simulink model "redundancy"  (R2020b)
settings: Solver=ode15s  StartTime=0.0  StopTime=T  MaxStep=0.01  RelTol=1e-3
values from neighbouring files (symbols this model uses):
  a1A = L1    (= 0.35)    [forward_kinematics_computation.m]
  a1B = L1    (= 0.35)    [forward_kinematics_computation.m]
  a2A = L2    (= 0.305)    [forward_kinematics_computation.m]
  a2B = L2    (= 0.305)    [forward_kinematics_computation.m]
  a3A = L3    (= 0.2662)    [forward_kinematics_computation.m]
  a3B = L3    (= 0.2662)    [forward_kinematics_computation.m]
  D = 1.047    [forward_kinematics_computation.m]
  dq0 = [0 0 0 0 0 0]'    [sim_redundancy.m]
  friction = [fv1p fv2p fv1A fv2A fv3A fv1B fv2B fv3B]    [sim_redundancy.m]
  g = [0 -g0 0]'    [sim_redundancy.m]
  Gd = diag([1000 1000 1000 1000 1000])    [sim_redundancy.m]
  Gd_nullspace = 10*eye(6)    [sim_redundancy.m]
  Gp = diag([3000 3000 3000 3000 1000])    [sim_redundancy.m]
  Gp_nullspace = 10*eye(6)    [sim_redundancy.m]
  info = struct('n_joints', n_joints,                'n_links', n_links,                'n_ee', n_ee,                'current_frame_index',    [1  2 3 4 5 6 7  8 9 10],                'previous_frame_index',   [0  1 2 3 4 2 6  7 5  8],                'next_frame_index',       [2 36 4 5 9 7 8 10 0  0],                'next_frame_type',        [0  1 0 0 0 0 0  0 0  0],                'previous_joint_index',  ...(+449 chars)    [sim_redundancy.m]
  Kd = 20*eye(6)    [sim_redundancy.m]
  Kp = 10*eye(6)    [sim_redundancy.m]
  L = 3.16 + 0.126    (= 3.286)    [forward_kinematics_computation.m]
  l1A = a1A/2    (= 0.175)    [forward_kinematics_computation.m]
  l1B = a1B/2    (= 0.175)    [forward_kinematics_computation.m]
  l2A = a2A/2    (= 0.1525)    [forward_kinematics_computation.m]
  l2B = a2B/2    (= 0.1525)    [forward_kinematics_computation.m]
  l3A = a3A/2    (= 0.1331)    [forward_kinematics_computation.m]
  l3B = a3B/2    (= 0.1331)    [forward_kinematics_computation.m]
  offA = -0.19    [forward_kinematics_computation.m]
  offB = 0.19    [forward_kinematics_computation.m]
  prova = 2    [sim_redundancy.m]
  q0 = [th1A_0 th2A_0 th3A_0 th1B_0 th2B_0 th3B_0]'    [sim_redundancy.m]
  qr = [0 -pi/3 pi/4 0 pi/4 pi/8]    [sim_redundancy.m]
  qr_ddot = zeros(1,6)    [sim_redundancy.m]
  qr_dot = zeros(1,6)    [sim_redundancy.m]
  th1A_0 = -pi/6    (= -0.523598775598)    [sim_redundancy.m]
  th1B_0 = pi/6    (= 0.523598775598)    [sim_redundancy.m]
  th2A_0 = pi/6    (= 0.523598775598)    [sim_redundancy.m]
  th2B_0 = -pi/6    (= -0.523598775598)    [sim_redundancy.m]
  th3A_0 = pi/6    (= 0.523598775598)    [sim_redundancy.m]
  th3B_0 = -pi/6    (= -0.523598775598)    [sim_redundancy.m]
  tipo_controllo = 1    [sim_redundancy.m]
  tipo_minimizzazione = 4    [sim_redundancy.m]
  x_ref = [-0.25 -0.8 0.19 -0.9 0]    [sim_redundancy.m]
  xddot_ref = [0 0 0 0 0]    [sim_redundancy.m]
  xdot_ref = [0 0 0 0 0]    [sim_redundancy.m]
undefined symbols (not defined in the file or in its folder): fv0, fv1A, fv1B, fv2A, fv2B, fv3A, fv3B, g0, Il1Azz, Il1Bzz, Il2Azz, Il2Bzz, Il3Azz, Il3Bzz, m_cables, m_crane, m_platform, ml1A, ml1B, ml2A, ml2B, ml3A, ml3B, X, Y, Z
libraries: sm_lib x137, nesl_utility x31
(part 5 of 5)

== matlab function redundancy/CLIK 2/Ja_dot*qd ==
  data: q input; qd input; out output; a1A parameter; a2A parameter; a3A parameter; a1B parameter; a2B parameter; a3B parameter; offA parameter; offB parameter; ml1A parameter; ml2A parameter; ml3A parameter; ml1B parameter; ml2B parameter; ml3B parameter; l1A parameter; l2A parameter; l3A parameter; l1B parameter; l2B parameter; l3B parameter
function out = fcn(q, qd, ...
                  a1A, a2A, a3A, a1B, a2B, a3B, offA, offB, ...
                  ml1A, ml2A, ml3A, ml1B, ml2B, ml3B, ...
                  l1A, l2A, l3A, l1B, l2B, l3B)

% Input
th1A = q(1);
th2A = q(2);
th3A = q(3);
th1B = q(4);
th2B = q(5);
th3B = q(6);
dth1A = qd(1);
dth2A = qd(2);
dth3A = qd(3);
dth1B = qd(4);
dth2B = qd(5);
dth3B = qd(6);

% Derivata dello Jacobiano
Jad = [                                                                                                                                  - a1A*dth1A*sin(th1A) - a3A*sin(th1A + th2A + th3A)*(dth1A + dth2A + dth3A) - a2A*sin(th1A + th2A)*(dth1A + dth2A),                                                                                - a3A*sin(th1A + th2A + th3A)*(dth1A + dth2A + dth3A) - a2A*sin(th1A + th2A)*(dth1A + dth2A),                                   -a3A*sin(th1A + th2A + th3A)*(dth1A + dth2A + dth3A),                                                                                                                                                                                                                                                    0,                                                                                                                                                                           0,                                                                                      0;
                                                                                                                                           a3A*cos(th1A + th2A + th3A)*(dth1A + dth2A + dth3A) + a2A*cos(th1A + th2A)*(dth1A + dth2A) + a1A*dth1A*cos(th1A),                                                                                  a3A*cos(th1A + th2A + th3A)*(dth1A + dth2A + dth3A) + a2A*cos(th1A + th2A)*(dth1A + dth2A),                                    a3A*cos(th1A + th2A + th3A)*(dth1A + dth2A + dth3A),                                                                                                                                                                                                                                                    0,                                                                                                                                                                           0,                                                                                      0;
                                                                                                                                                                                                                                                          0,                                                                                                                                                                           0,                                                                                      0,                                                                                                                                   - a1B*dth1B*sin(th1B) - a3B*sin(th1B + th2B + th3B)*(dth1B + dth2B + dth3B) - a2B*sin(th1B + th2B)*(dth1B + dth2B),                                                                                - a3B*sin(th1B + th2B + th3B)*(dth1B + dth2B + dth3B) - a2B*sin(th1B + th2B)*(dth1B + dth2B),                                   -a3B*sin(th1B + th2B + th3B)*(dth1B + dth2B + dth3B);
                                                                                                                                                                                                                                                          0,                                                                                                                                                                           0,                                                                                      0,                                                                                                                                     a3B*cos(th1B + th2B + th3B)*(dth1B + dth2B + dth3B) + a2B*cos(th1B + th2B)*(dth1B + dth2B) + a1B*dth1B*cos(th1B),                                                                                  a3B*cos(th1B + th2B + th3B)*(dth1B + dth2B + dth3B) + a2B*cos(th1B + th2B)*(dth1B + dth2B),                                    a3B*cos(th1B + th2B + th3B)*(dth1B + dth2B + dth3B);
       -(ml3A*(a1A*dth1A*sin(th1A) + l3A*sin(th1A + th2A + th3A)*(dth1A + dth2A + dth3A) + a2A*sin(th1A + th2A)*(dth1A + dth2A)) + ml2A*(a1A*dth1A*sin(th1A) + l2A*sin(th1A + th2A)*(dth1A + dth2A)) + dth1A*l1A*ml1A*sin(th1A))/(2*ml1A + 2*ml2A + 2*ml3A), -(ml3A*(l3A*sin(th1A + th2A + th3A)*(dth1A + dth2A + dth3A) + a2A*sin(th1A + th2A)*(dth1A + dth2A)) + l2A*ml2A*sin(th1A + th2A)*(dth1A + dth2A))/(2*ml1A + 2*ml2A + 2*ml3A), -(l3A*ml3A*sin(th1A + th2A + th3A)*(dth1A + dth2A + dth3A))/(2*ml1A + 2*ml2A + 2*ml3A), -(ml3B*(a1B*dth1B*sin(th1B) + l3B*sin(th1B + th2B + th3B)*(dth1B + dth2B + dth3B) + a2B*sin(th1B + th2B)*(dth1B + dth2B)) + ml2B*(a1B*dth1B*sin(th1B) + l2B*sin(th1B + th2B)*(dth1B + dth2B)) + dth1B*l1B*ml1B*sin(th1B))/(2*ml1B + 2*ml2B + 2*ml3B), -(ml3B*(l3B*sin(th1B + th2B + th3B)*(dth1B + dth2B + dth3B) + a2B*sin(th1B + th2B)*(dth1B + dth2B)) + l2B*ml2B*sin(th1B + th2B)*(dth1B + dth2B))/(2*ml1B + 2*ml2B + 2*ml3B), -(l3B*ml3B*sin(th1B + th2B + th3B)*(dth1B + dth2B + dth3B))/(2*ml1B + 2*ml2B + 2*ml3B)];

out = Jad*qd;

end

== matlab function redundancy/CLIK 1/Controller ==
  data: in input; q input; qd input; a1A parameter; a2A parameter; a3A parameter; a1B parameter; a2B parameter; a3B parameter; y output; offA parameter; offB parameter; Gd_nullspace parameter; Gp_nullspace parameter; q0 parameter
function y  = fcn(in, q, qd, ...
                  a1A, a2A, a3A, a1B, a2B, a3B, offA, offB, ...
                  Gd_nullspace, Gp_nullspace, q0)

% Input
th1A = q(1);
th2A = q(2);
th3A = q(3);
th1B = q(4);
th2B = q(5);
th3B = q(6);

% Jacobiano
Ja = [a2A*cos(th1A + th2A) + a1A*cos(th1A) + a3A*cos(th1A + th2A + th3A), a2A*cos(th1A + th2A) + a3A*cos(th1A + th2A + th3A), a3A*cos(th1A + th2A + th3A),                                                                  0,                                                  0,                           0;
      a2A*sin(th1A + th2A) + a1A*sin(th1A) + a3A*sin(th1A + th2A + th3A), a2A*sin(th1A + th2A) + a3A*sin(th1A + th2A + th3A), a3A*sin(th1A + th2A + th3A),                                                                  0,                                                  0,                           0;
                                                                       0,                                                  0,                           0, a2B*cos(th1B + th2B) + a1B*cos(th1B) + a3B*cos(th1B + th2B + th3B), a2B*cos(th1B + th2B) + a3B*cos(th1B + th2B + th3B), a3B*cos(th1B + th2B + th3B);
                                                                       0,                                                  0,                           0, a2B*sin(th1B + th2B) + a1B*sin(th1B) + a3B*sin(th1B + th2B + th3B), a2B*sin(th1B + th2B) + a3B*sin(th1B + th2B + th3B), a3B*sin(th1B + th2B + th3B)];

% Control
y = pinv(Ja)*in + (eye(6)-pinv(Ja)*Ja)*(Gd_nullspace*(-qd)+Gp_nullspace*(q0-q));

end

== matlab function redundancy/CLIK 1/Direct Kinematics ==
  data: q input; xe output; a1A parameter; a2A parameter; a3A parameter; a1B parameter; a2B parameter; a3B parameter; offA parameter; offB parameter
function xe = fcn(q, ...
                  a1A, a2A, a3A, a1B, a2B, a3B, offA, offB)

% Input
th1A = q(1);
th2A = q(2);
th3A = q(3);
th1B = q(4);
th2B = q(5);
th3B = q(6);

% Cinematica diretta
xe = [ offA + a1A*sin(th1A) + a2A*sin(th1A + th2A) + a3A*sin(th1A + th2A + th3A);
            - a1A*cos(th1A) - a2A*cos(th1A + th2A) - a3A*cos(th1A + th2A + th3A);
       offB + a1B*sin(th1B) + a2B*sin(th1B + th2B) + a3B*sin(th1B + th2B + th3B);
            - a1B*cos(th1B) - a2B*cos(th1B + th2B) - a3B*cos(th1B + th2B + th3B)];

end

== matlab function redundancy/CLIK 1/Ja*qd ==
  data: q input; qd input; xe_dot output; a1A parameter; a2A parameter; a3A parameter; a1B parameter; a2B parameter; a3B parameter
function xe_dot = fcn(q, qd, ...
                      a1A, a2A, a3A, a1B, a2B, a3B)

% Input
th1A = q(1);
th2A = q(2);
th3A = q(3);
th1B = q(4);
th2B = q(5);
th3B = q(6);

% Jacobiano
Ja = [a2A*cos(th1A + th2A) + a1A*cos(th1A) + a3A*cos(th1A + th2A + th3A), a2A*cos(th1A + th2A) + a3A*cos(th1A + th2A + th3A), a3A*cos(th1A + th2A + th3A),                                                                  0,                                                  0,                           0;
      a2A*sin(th1A + th2A) + a1A*sin(th1A) + a3A*sin(th1A + th2A + th3A), a2A*sin(th1A + th2A) + a3A*sin(th1A + th2A + th3A), a3A*sin(th1A + th2A + th3A),                                                                  0,                                                  0,                           0;
                                                                       0,                                                  0,                           0, a2B*cos(th1B + th2B) + a1B*cos(th1B) + a3B*cos(th1B + th2B + th3B), a2B*cos(th1B + th2B) + a3B*cos(th1B + th2B + th3B), a3B*cos(th1B + th2B + th3B);
                                                                       0,                                                  0,                           0, a2B*sin(th1B + th2B) + a1B*sin(th1B) + a3B*sin(th1B + th2B + th3B), a2B*sin(th1B + th2B) + a3B*sin(th1B + th2B + th3B), a3B*sin(th1B + th2B + th3B)];

xe_dot = Ja*qd;

end

== matlab function redundancy/CLIK 1/Ja_dot*qd ==
  data: q input; qd input; out output; a1A parameter; a2A parameter; a3A parameter; a1B parameter; a2B parameter; a3B parameter
function out = fcn(q, qd, ...
                   a1A, a2A, a3A, a1B, a2B, a3B)

% Input
th1A = q(1);
th2A = q(2);
th3A = q(3);
th1B = q(4);
th2B = q(5);
th3B = q(6);
dth1A = qd(1);
dth2A = qd(2);
dth3A = qd(3);
dth1B = qd(4);
dth2B = qd(5);
dth3B = qd(6);

% Derivata dello Jacobiano
Jad = [- a1A*dth1A*sin(th1A) - a3A*sin(th1A + th2A + th3A)*(dth1A + dth2A + dth3A) - a2A*sin(th1A + th2A)*(dth1A + dth2A), - a3A*sin(th1A + th2A + th3A)*(dth1A + dth2A + dth3A) - a2A*sin(th1A + th2A)*(dth1A + dth2A), -a3A*sin(th1A + th2A + th3A)*(dth1A + dth2A + dth3A),                                                                                                                  0,                                                                                            0,                                                    0;
         a3A*cos(th1A + th2A + th3A)*(dth1A + dth2A + dth3A) + a2A*cos(th1A + th2A)*(dth1A + dth2A) + a1A*dth1A*cos(th1A),   a3A*cos(th1A + th2A + th3A)*(dth1A + dth2A + dth3A) + a2A*cos(th1A + th2A)*(dth1A + dth2A),  a3A*cos(th1A + th2A + th3A)*(dth1A + dth2A + dth3A),                                                                                                                  0,                                                                                            0,                                                    0;
                                                                                                                        0,                                                                                            0,                                                    0, - a1B*dth1B*sin(th1B) - a3B*sin(th1B + th2B + th3B)*(dth1B + dth2B + dth3B) - a2B*sin(th1B + th2B)*(dth1B + dth2B), - a3B*sin(th1B + th2B + th3B)*(dth1B + dth2B + dth3B) - a2B*sin(th1B + th2B)*(dth1B + dth2B), -a3B*sin(th1B + th2B + th3B)*(dth1B + dth2B + dth3B);
                                                                                                                        0,                                                                                            0,                                                    0,   a3B*cos(th1B + th2B + th3B)*(dth1B + dth2B + dth3B) + a2B*cos(th1B + th2B)*(dth1B + dth2B) + a1B*dth1B*cos(th1B),   a3B*cos(th1B + th2B + th3B)*(dth1B + dth2B + dth3B) + a2B*cos(th1B + th2B)*(dth1B + dth2B),  a3B*cos(th1B + th2B + th3B)*(dth1B + dth2B + dth3B)];

out = Jad*qd;

end

== matlab function redundancy/CLIK 3/Controller1 ==
  data: in input; q input; qd input; a1A parameter; a2A parameter; a3A parameter; a1B parameter; a2B parameter; a3B parameter; g0 parameter; Il1Azz parameter; Il2Azz parameter; Il3Azz parameter; Il1Bzz parameter; Il2Bzz parameter; Il3Bzz parameter; y output; fv1A parameter; fv2A parameter; fv3A parameter; fv1B parameter; fv2B parameter; fv3B parameter; ml1A parameter; ml2A parameter; ml3A parameter; ml1B parameter; ml2B parameter; ml3B parameter; l1A parameter; l2A parameter; l3A parameter; l1B parameter; l2B parameter; l3B parameter; prova parameter; tipo_minimizzazione parameter; fv0 parameter; offA parameter; offB parameter
function y  = fcn(in, q, qd, ...
                   a1A, a2A, a3A, a1B, a2B, a3B, g0,...
                   Il1Azz, Il2Azz, Il3Azz, Il1Bzz, Il2Bzz, Il3Bzz, ...
                   fv1A, fv2A, fv3A, fv1B, fv2B, fv3B, ...
                   ml1A, ml2A, ml3A, ml1B, ml2B, ml3B, ...
                   l1A, l2A, l3A, l1B, l2B, l3B, prova, tipo_minimizzazione, fv0, offA, offB)

% Input
th1A = q(1);
th2A = q(2);
th3A = q(3);
th1B = q(4);
th2B = q(5);
th3B = q(6);
dth1A = qd(1);
dth2A = qd(2);
dth3A = qd(3);
dth1B = qd(4);
dth2B = qd(5);
dth3B = qd(6);

% Matrice B
B = [ Il1Azz + Il2Azz + Il3Azz + a1A^2*ml2A + a1A^2*ml3A + a2A^2*ml3A + l1A^2*ml1A + l2A^2*ml2A + l3A^2*ml3A + 2*a1A*l3A*ml3A*cos(th2A + th3A) + 2*a1A*a2A*ml3A*cos(th2A) + 2*a1A*l2A*ml2A*cos(th2A) + 2*a2A*l3A*ml3A*cos(th3A), ml3A*a2A^2 + 2*ml3A*cos(th3A)*a2A*l3A + a1A*ml3A*cos(th2A)*a2A + ml2A*l2A^2 + a1A*ml2A*cos(th2A)*l2A + ml3A*l3A^2 + a1A*ml3A*cos(th2A + th3A)*l3A + Il2Azz + Il3Azz, Il3Azz + l3A^2*ml3A + a1A*l3A*ml3A*cos(th2A + th3A) + a2A*l3A*ml3A*cos(th3A),                                                                                                                                                                                                                         0,                                                                                                                                                                   0,                                                                                                                                                                                     0;
                                                            ml3A*a2A^2 + 2*ml3A*cos(th3A)*a2A*l3A + a1A*ml3A*cos(th2A)*a2A + ml2A*l2A^2 + a1A*ml2A*cos(th2A)*l2A + ml3A*l3A^2 + a1A*ml3A*cos(th2A + th3A)*l3A + Il2Azz + Il3Azz,                                                                                   ml3A*a2A^2 + 2*ml3A*cos(th3A)*a2A*l3A + ml2A*l2A^2 + ml3A*l3A^2 + Il2Azz + Il3Azz,                                 ml3A*l3A^2 + a2A*ml3A*cos(th3A)*l3A + Il3Azz,                                                                                                                                                                                                                         0,                                                                                                                                                                   0,                                                                                                                                                                                     0;
                                                                                                                                                   Il3Azz + l3A^2*ml3A + a1A*l3A*ml3A*cos(th2A + th3A) + a2A*l3A*ml3A*cos(th3A),                                                                                                                        ml3A*l3A^2 + a2A*ml3A*cos(th3A)*l3A + Il3Azz,                                                          ml3A*l3A^2 + Il3Azz,                                                                                                                                                                                                                         0,                                                                                                                                                                   0,                                                                                                                                                                                     0;
                                                                                                                                                                                                                              0,                                                                                                                                                                   0,                                                                            0, Il1Bzz + Il2Bzz + Il3Bzz + a2A^2*ml3B + a1B^2*ml2B + a1B^2*ml3B + l1B^2*ml1B + l2B^2*ml2B + l3B^2*ml3B + 2*a1B*l3B*ml3B*cos(th2B + th3B) + 2*a2A*a1B*ml3B*cos(th2B) + 2*a2A*l3B*ml3B*cos(th3B) + 2*a1B*l2B*ml2B*cos(th2B), ml3B*a2A^2 + 2*ml3B*cos(th3B)*a2A*l3B + a1B*ml3B*cos(th2B)*a2A + ml2B*l2B^2 + a1B*ml2B*cos(th2B)*l2B + ml3B*l3B^2 + a1B*ml3B*cos(th2B + th3B)*l3B + Il2Bzz + Il3Bzz, Il3Bzz + a2A^2*ml3B + l3B^2*ml3B - a2A*a2B*ml3B + a1B*l3B*ml3B*cos(th2B + th3B) + a2A*a1B*ml3B*cos(th2B) - a1B*a2B*ml3B*cos(th2B) + 2*a2A*l3B*ml3B*cos(th3B) - a2B*l3B*ml3B*cos(th3B);
                                                                                                                                                                                                                              0,                                                                                                                                                                   0,                                                                            0,                                                       ml3B*a2A^2 + 2*ml3B*cos(th3B)*a2A*l3B + a1B*ml3B*cos(th2B)*a2A + ml2B*l2B^2 + a1B*ml2B*cos(th2B)*l2B + ml3B*l3B^2 + a1B*ml3B*cos(th2B + th3B)*l3B + Il2Bzz + Il3Bzz,                                                                                   ml3B*a2A^2 + 2*ml3B*cos(th3B)*a2A*l3B + ml2B*l2B^2 + ml3B*l3B^2 + Il2Bzz + Il3Bzz,                                                                                   ml3B*a2A^2 + 2*ml3B*cos(th3B)*a2A*l3B - a2B*ml3B*a2A + ml3B*l3B^2 - a2B*ml3B*cos(th3B)*l3B + Il3Bzz;
                                                                                                                                                                                                                              0,                                                                                                                                                                   0,                                                                            0,                                     Il3Bzz + a2A^2*ml3B + l3B^2*ml3B - a2A*a2B*ml3B + a1B*l3B*ml3B*cos(th2B + th3B) + a2A*a1B*ml3B*cos(th2B) - a1B*a2B*ml3B*cos(th2B) + 2*a2A*l3B*ml3B*cos(th3B) - a2B*l3B*ml3B*cos(th3B),                                                                 ml3B*a2A^2 + 2*ml3B*cos(th3B)*a2A*l3B - a2B*ml3B*a2A + ml3B*l3B^2 - a2B*ml3B*cos(th3B)*l3B + Il3Bzz,                                                                  ml3B*a2A^2 - 2*ml3B*a2A*a2B + 2*ml3B*cos(th3B)*a2A*l3B + ml3B*a2B^2 - 2*ml3B*cos(th3B)*a2B*l3B + ml3B*l3B^2 + Il3Bzz];

% Matrice C
C = [ - dth2A*(a1A*l3A*ml3A*sin(th2A + th3A) + a1A*a2A*ml3A*sin(th2A) + a1A*l2A*ml2A*sin(th2A)) - dth3A*(a1A*l3A*ml3A*sin(th2A + th3A) + a2A*l3A*ml3A*sin(th3A)), - a1A*dth1A*(a2A*ml3A*sin(th2A) + l2A*ml2A*sin(th2A) + l3A*ml3A*sin(th2A + th3A)) - a1A*dth2A*(a2A*ml3A*sin(th2A) + l2A*ml2A*sin(th2A) + l3A*ml3A*sin(th2A + th3A)) - dth3A*l3A*ml3A*(a1A*sin(th2A + th3A) + a2A*sin(th3A)), -l3A*ml3A*(a1A*sin(th2A + th3A) + a2A*sin(th3A))*(dth1A + dth2A + dth3A),                                                                                                                                                                 0,                                                                                                                                                                                                                                                                                  0,                                                                                                                                                                                                                                                0;
                                          dth1A*(a1A*l3A*ml3A*sin(th2A + th3A) + a1A*a2A*ml3A*sin(th2A) + a1A*l2A*ml2A*sin(th2A)) - a2A*dth3A*l3A*ml3A*sin(th3A),                                                                                                                                                                                               -a2A*dth3A*l3A*ml3A*sin(th3A),                          -a2A*l3A*ml3A*sin(th3A)*(dth1A + dth2A + dth3A),                                                                                                                                                                 0,                                                                                                                                                                                                                                                                                  0,                                                                                                                                                                                                                                                0;
                                                                   dth1A*(a1A*l3A*ml3A*sin(th2A + th3A) + a2A*l3A*ml3A*sin(th3A)) + a2A*dth2A*l3A*ml3A*sin(th3A),                                                                                                                                                                                      a2A*l3A*ml3A*sin(th3A)*(dth1A + dth2A),                                                                        0,                                                                                                                                                                 0,                                                                                                                                                                                                                                                                                  0,                                                                                                                                                                                                                                                0;
                                                                                                                                                               0,                                                                                                                                                                                                                           0,                                                                        0,        - dth2B*(a1B*l3B*ml3B*sin(th2B + th3B) + a2A*a1B*ml3B*sin(th2B) + a1B*l2B*ml2B*sin(th2B)) - dth3B*(a1B*l3B*ml3B*sin(th2B + th3B) + a2A*l3B*ml3B*sin(th3B)), - 0.5000*dth3B*ml3B*(a2A*a1B*sin(th2B) - a1B*a2B*sin(th2B) + 2*a2A*l3B*sin(th3B) + 2*a1B*l3B*sin(th2B + th3B)) - a1B*dth1B*(a2A*ml3B*sin(th2B) + l2B*ml2B*sin(th2B) + l3B*ml3B*sin(th2B + th3B)) - a1B*dth2B*(a2A*ml3B*sin(th2B) + l2B*ml2B*sin(th2B) + l3B*ml3B*sin(th2B + th3B)), - 0.5000*dth2B*ml3B*(a2A*a1B*sin(th2B) - a1B*a2B*sin(th2B) + 2*a2A*l3B*sin(th3B) + 2*a1B*l3B*sin(th2B + th3B)) - dth1B*l3B*ml3B*(a1B*sin(th2B + th3B) + a2A*sin(th3B)) - dth3B*l3B*ml3B*(a1B*sin(th2B + th3B) + 2*a2A*sin(th3B) - a2B*sin(th3B));
                                                                                                                                                               0,                                                                                                                                                                                                                           0,                                                                        0, a1B*dth1B*(a2A*ml3B*sin(th2B) + l2B*ml2B*sin(th2B) + l3B*ml3B*sin(th2B + th3B)) - 0.5000*dth3B*ml3B*(a1B*a2B*sin(th2B) - a2A*a1B*sin(th2B) + 2*a2A*l3B*sin(th3B)),                                                                                                                                                                                                                                                      -a2A*dth3B*l3B*ml3B*sin(th3B),                                                      - dth1B*(0.5000*a1B*a2B*ml3B*sin(th2B) - 0.5000*a2A*a1B*ml3B*sin(th2B) + a2A*l3B*ml3B*sin(th3B)) - dth3B*(2*a2A*l3B*ml3B*sin(th3B) - a2B*l3B*ml3B*sin(th3B)) - a2A*dth2B*l3B*ml3B*sin(th3B);
                                                                                                                                                               0,                                                                                                                                                                                                                           0,                                                                        0,   dth2B*(0.5000*a1B*a2B*ml3B*sin(th2B) - 0.5000*a2A*a1B*ml3B*sin(th2B) + a2A*l3B*ml3B*sin(th3B)) + dth1B*(a1B*l3B*ml3B*sin(th2B + th3B) + a2A*l3B*ml3B*sin(th3B)),                                                                                                                                                      dth1B*(0.5000*a1B*a2B*ml3B*sin(th2B) - 0.5000*a2A*a1B*ml3B*sin(th2B) + a2A*l3B*ml3B*sin(th3B)) + a2A*dth2B*l3B*ml3B*sin(th3B),                                                                                                                                                                                                            -dth3B*l3B*ml3B*sin(th3B)*(a2A - a2B)];

% Matrice Fv
Fv = diag([fv1A fv2A fv3A fv1B fv2B fv3B]);

% Vettore g 
g = [- g0*ml3A*(a2A*cos(th1A + th2A) + a1A*cos(th1A) + l3A*cos(th1A + th2A + th3A)) - g0*ml2A*(l2A*cos(th1A + th2A) + a1A*cos(th1A)) - g0*l1A*ml1A*cos(th1A);
     - g0*ml3A*(a2A*cos(th1A + th2A) + l3A*cos(th1A + th2A + th3A)) - g0*l2A*ml2A*cos(th1A + th2A);
     - g0*l3A*ml3A*cos(th1A + th2A + th3A);
     - g0*ml3B*(a2A*cos(th1B + th2B) + a1B*cos(th1B) + l3B*cos(th1B + th2B + th3B)) - g0*ml2B*(l2B*cos(th1B + th2B) + a1B*cos(th1B)) - g0*l1B*ml1B*cos(th1B);
     - g0*ml3B*(a2A*cos(th1B + th2B) + l3B*cos(th1B + th2B + th3B)) - g0*l2B*ml2B*cos(th1B + th2B);
     - g0*ml3B*(a2A*cos(th1B + th2B) - a2B*cos(th1B + th2B) + l3B*cos(th1B + th2B + th3B))];
 
n = C*qd + Fv*qd + g;

Ja = [                                                                                                - a2A*sin(th1A + th2A) - a1A*sin(th1A) - a3A*sin(th1A + th2A + th3A),                                                          - a2A*sin(th1A + th2A) - a3A*sin(th1A + th2A + th3A),                             -a3A*sin(th1A + th2A + th3A),                                                                                                                                                                    0,                                                                                                             0,                                                        0; 
                                                                                                        a2A*cos(th1A + th2A) + a1A*cos(th1A) + a3A*cos(th1A + th2A + th3A),                                                            a2A*cos(th1A + th2A) + a3A*cos(th1A + th2A + th3A),                              a3A*cos(th1A + th2A + th3A),                                                                                                                                                                    0,                                                                                                             0,                                                        0;
                                                                                                                                                                         0,                                                                                                             0,                                                        0,                                                                                                 - a2B*sin(th1B + th2B) - a1B*sin(th1B) - a3B*sin(th1B + th2B + th3B),                                                          - a2B*sin(th1B + th2B) - a3B*sin(th1B + th2B + th3B),                             -a3B*sin(th1B + th2B + th3B);
                                                                                                                                                                         0,                                                                                                             0,                                                        0,                                                                                                   a2B*cos(th1B + th2B) + a1B*cos(th1B) + a3B*cos(th1B + th2B + th3B),                                                            a2B*cos(th1B + th2B) + a3B*cos(th1B + th2B + th3B),                              a3B*cos(th1B + th2B + th3B);
      -(ml3A*(a2A*sin(th1A + th2A) + a1A*sin(th1A) + l3A*sin(th1A + th2A + th3A)) + ml2A*(l2A*sin(th1A + th2A) + a1A*sin(th1A)) + l1A*ml1A*sin(th1A))/(ml1A + ml2A + ml3A), -(ml3A*(a2A*sin(th1A + th2A) + l3A*sin(th1A + th2A + th3A)) + l2A*ml2A*sin(th1A + th2A))/(ml1A + ml2A + ml3A), -(l3A*ml3A*sin(th1A + th2A + th3A))/(ml1A + ml2A + ml3A), -(ml3B*(a2B*sin(th1B + th2B) + a1B*sin(th1B) + l3B*sin(th1B + th2B + th3B)) + ml2B*(l2B*sin(th1B + th2B) + a1B*sin(th1B)) + l1B*ml1B*sin(th1B))/(ml1B + ml2B + ml3B), -(ml3B*(a2B*sin(th1B + th2B) + l3B*sin(th1B + th2B + th3B)) + l2B*ml2B*sin(th1B + th2B))/(ml1B + ml2B + ml3B), -(l3B*ml3B*sin(th1B + th2B + th3B))/(ml1B + ml2B + ml3B)];

% Matrix for controller
P = eye(6)-pinv(Ja)*Ja;

%% f1Ax
M_11A =  - a1A*ml2A*sin(th1A) - a1A*ml3A*sin(th1A) - l1A*ml1A*sin(th1A) - a2A*ml3A*sin(th1A + th2A) - l2A*ml2A*sin(th1A + th2A) - l3A*ml3A*sin(th1A + th2A + th3A);
M_12A =  - a2A*ml3A*sin(th1A + th2A) - l2A*ml2A*sin(th1A + th2A) - l3A*ml3A*sin(th1A + th2A + th3A);
M_13A =  - l3A*ml3A*sin(th1A + th2A + th3A);
M1A = [M_11A, M_12A, M_13A];
m1A =  - a1A*dth1A^2*ml2A*cos(th1A) - a1A*dth1A^2*ml3A*cos(th1A) - dth1A^2*l1A*ml1A*cos(th1A) - 2*a2A*dth1A*dth2A*ml3A*cos(th1A + th2A) - 2*dth1A*dth2A*l2A*ml2A*cos(th1A + th2A)...
      - a2A*dth1A^2*ml3A*cos(th1A + th2A) - a2A*dth2A^2*ml3A*cos(th1A + th2A) - dth1A^2*l2A*ml2A*cos(th1A + th2A) - dth2A^2*l2A*ml2A*cos(th1A + th2A) - dth1A^2*l3A*ml3A*cos(th1A + th2A + th3A) ...
      - dth2A^2*l3A*ml3A*cos(th1A + th2A + th3A) - dth3A^2*l3A*ml3A*cos(th1A + th2A + th3A) - 2*dth1A*dth2A*l3A*ml3A*cos(th1A + th2A + th3A) - 2*dth1A*dth3A*l3A*ml3A*cos(th1A + th2A + th3A) ...
      - 2*dth2A*dth3A*l3A*ml3A*cos(th1A + th2A + th3A);
 
% f1Bx
M_11B =  - a1B*ml2B*sin(th1B) - a1B*ml3B*sin(th1B) - l1B*ml1B*sin(th1B) - a2B*ml3B*sin(th1B + th2B) - l2B*ml2B*sin(th1B + th2B) - l3B*ml3B*sin(th1B + th2B + th3B);
M_12B =  - a2B*ml3B*sin(th1B + th2B) - l2B*ml2B*sin(th1B + th2B) - l3B*ml3B*sin(th1B + th2B + th3B);
M_13B =  - l3B*ml3B*sin(th1B + th2B + th3B);
M1B = [M_11B, M_12B, M_13B];
m1B =  - a1B*dth1B^2*ml2B*cos(th1B) - a1B*dth1B^2*ml3B*cos(th1B) - dth1B^2*l1B*ml1B*cos(th1B) - 2*a2B*dth1B*dth2B*ml3B*cos(th1B + th2B) - 2*dth1B*dth2B*l2B*ml2B*cos(th1B + th2B)...
      - a2B*dth1B^2*ml3B*cos(th1B + th2B) - a2B*dth2B^2*ml3B*cos(th1B + th2B) - dth1B^2*l2B*ml2B*cos(th1B + th2B) - dth2B^2*l2B*ml2B*cos(th1B + th2B) - dth1B^2*l3B*ml3B*cos(th1B + th2B + th3B) ...
      - dth2B^2*l3B*ml3B*cos(th1B + th2B + th3B) - dth3B^2*l3B*ml3B*cos(th1B + th2B + th3B) - 2*dth1B*dth2B*l3B*ml3B*cos(th1B + th2B + th3B) - 2*dth1B*dth3B*l3B*ml3B*cos(th1B + th2B + th3B) ...
      - 2*dth2B*dth3B*l3B*ml3B*cos(th1B + th2B + th3B);

%% f1Ay
M_21A = a1A*ml2A*cos(th1A) + a1A*ml3A*cos(th1A) + l1A*ml1A*cos(th1A) + a2A*ml3A*cos(th1A + th2A) + l2A*ml2A*cos(th1A + th2A) + l3A*ml3A*cos(th1A + th2A + th3A);
M_22A = a2A*ml3A*cos(th1A + th2A) + l2A*ml2A*cos(th1A + th2A) + l3A*ml3A*cos(th1A + th2A + th3A);
M_23A = l3A*ml3A*cos(th1A + th2A + th3A);
M2A = [M_21A, M_22A, M_23A];
m2A = - dth1A^2*l3A*ml3A*sin(th1A + th2A + th3A) - dth2A^2*l3A*ml3A*sin(th1A + th2A + th3A) - dth3A^2*l3A*ml3A*sin(th1A + th2A + th3A) - a2A*dth1A^2*ml3A*sin(th1A + th2A) ...
      - a2A*dth2A^2*ml3A*sin(th1A + th2A) - dth1A^2*l2A*ml2A*sin(th1A + th2A) - dth2A^2*l2A*ml2A*sin(th1A + th2A) - a1A*dth1A^2*ml2A*sin(th1A) - a1A*dth1A^2*ml3A*sin(th1A) ...
      - dth1A^2*l1A*ml1A*sin(th1A) - 2*dth1A*dth2A*l3A*ml3A*sin(th1A + th2A + th3A) - 2*dth1A*dth3A*l3A*ml3A*sin(th1A + th2A + th3A) - 2*dth2A*dth3A*l3A*ml3A*sin(th1A + th2A + th3A) ...
      - 2*a2A*dth1A*dth2A*ml3A*sin(th1A + th2A) - 2*dth1A*dth2A*l2A*ml2A*sin(th1A + th2A);

% f1By
M_21B = a1B*ml2B*cos(th1B) + a1B*ml3B*cos(th1B) + l1B*ml1B*cos(th1B) + a2B*ml3B*cos(th1B + th2B) + l2B*ml2B*cos(th1B + th2B) + l3B*ml3B*cos(th1B + th2B + th3B);
M_22B = a2B*ml3B*cos(th1B + th2B) + l2B*ml2B*cos(th1B + th2B) + l3B*ml3B*cos(th1B + th2B + th3B);
M_23B = l3B*ml3B*cos(th1B + th2B + th3B);
M2B = [M_21B, M_22B, M_23B];
m2B = - dth1B^2*l3B*ml3B*sin(th1B + th2B + th3B) - dth2B^2*l3B*ml3B*sin(th1B + th2B + th3B) - dth3B^2*l3B*ml3B*sin(th1B + th2B + th3B) - a2B*dth1B^2*ml3B*sin(th1B + th2B) ...
      - a2B*dth2B^2*ml3B*sin(th1B + th2B) - dth1B^2*l2B*ml2B*sin(th1B + th2B) - dth2B^2*l2B*ml2B*sin(th1B + th2B) - a1B*dth1B^2*ml2B*sin(th1B) - a1B*dth1B^2*ml3B*sin(th1B) ...
      - dth1B^2*l1B*ml1B*sin(th1B) - 2*dth1B*dth2B*l3B*ml3B*sin(th1B + th2B + th3B) - 2*dth1B*dth3B*l3B*ml3B*sin(th1B + th2B + th3B) - 2*dth2B*dth3B*l3B*ml3B*sin(th1B + th2B + th3B) ...
      - 2*a2B*dth1B*dth2B*ml3B*sin(th1B + th2B) - 2*dth1B*dth2B*l2B*ml2B*sin(th1B + th2B);

%%
if tipo_minimizzazione == 1 % (Minimizzazione forza orizzontale)
    if prova == 1                       % (Minimizzazione f1Ax e f1Bx separatamente)
        M = [       M1A, zeros(1,3);
             zeros(1,3),       M1B];
        m = [m1A; 
             m1B];
    else                                % (Minimizzazione somma f1Ax e f1Bx (resta un gdl libero))
        M = [M1A, M1B];
        m = m1A + m1B;
    end
elseif tipo_minimizzazione == 2 % (Minimizzazione forza verticale)
    if prova == 1                       % (Minimizzazione f1Ay e f1By separatamente)
        M = [       M2A, zeros(1,3);
             zeros(1,3),       M2B];
        m = [m2A; 
             m2B];
    else                                % (Minimizzazione somma f1Ay e f1By (resta un gdl libero))
        M = [M2A, M2B];
        m = m2A + m2B;
    end    
else % (Minimizzazione forza orizzontale e verticale contemporaneamente)
    M = [M1A, M1B;
         M2A, M2B];
    m = [m1A+m1B; 
         m2A+m2B];    
end

% Control
y = pinv(Ja)*in - pinv(M*P)*(M*pinv(Ja)*in+m);

end

== matlab function redundancy/CLIK 3/Direct Kinematics ==
  data: q input; xe output; a1A parameter; a2A parameter; a3A parameter; a1B parameter; a2B parameter; a3B parameter; offA parameter; offB parameter; ml1A parameter; ml2A parameter; ml3A parameter; ml1B parameter; ml2B parameter; ml3B parameter; l1A parameter; l2A parameter; l3A parameter; l1B parameter; l2B parameter; l3B parameter
function xe = fcn(q, ...
                  a1A, a2A, a3A, a1B, a2B, a3B, offA, offB, ...
                  ml1A, ml2A, ml3A, ml1B, ml2B, ml3B, ...
                  l1A, l2A, l3A, l1B, l2B, l3B)

% Input
th1A = q(1);
th2A = q(2);
th3A = q(3);
th1B = q(4);
th2B = q(5);
th3B = q(6);
       
% Center of Mass of the arms
pl1A = [offA+l1A*sin(th1A), -l1A*cos(th1A)]';
pl2A = [offA+a1A*sin(th1A)+l2A*sin(th1A+th2A), -a1A*cos(th1A)-l2A*cos(th1A+th2A)]';
pl3A = [offA+a1A*sin(th1A)+a2A*sin(th1A+th2A)+l3A*sin(th1A+th2A+th3A), -a1A*cos(th1A)-a2A*cos(th1A+th2A)-l3A*cos(th1A+th2A+th3A)]';
pl1B = [offB+l1B*sin(th1B), -l1B*cos(th1B)]';
pl2B = [offB+a1B*sin(th1B)+l2B*sin(th1B+th2B), -a1B*cos(th1B)-l2B*cos(th1B+th2B)]';
pl3B = [offB+a1B*sin(th1B)+a2B*sin(th1B+th2B)+l3B*sin(th1B+th2B+th3B), -a1B*cos(th1B)-a2B*cos(th1B+th2B)-l3B*cos(th1B+th2B+th3B)]';

cmxA = (ml1A*pl1A(1)+ml2A*pl2A(1)+ml3A*pl3A(1))/(ml1A+ml2A+ml3A);
cmyA = (ml1A*pl1A(2)+ml2A*pl2A(2)+ml3A*pl3A(2))/(ml1A+ml2A+ml3A);
cmxB = (ml1B*pl1B(1)+ml2B*pl2B(1)+ml3B*pl3B(1))/(ml1B+ml2B+ml3B);
cmyB = (ml1B*pl1B(2)+ml2B*pl2B(2)+ml3B*pl3B(2))/(ml2B+ml2B+ml3B);
cmx = (cmxA + cmxB)/2;

% Cinematica diretta
xe = [ offA + a1A*sin(th1A) + a2A*sin(th1A + th2A) + a3A*sin(th1A + th2A + th3A);
            - a1A*cos(th1A) - a2A*cos(th1A + th2A) - a3A*cos(th1A + th2A + th3A);
       offB + a1B*sin(th1B) + a2B*sin(th1B + th2B) + a3B*sin(th1B + th2B + th3B);
            - a1B*cos(th1B) - a2B*cos(th1B + th2B) - a3B*cos(th1B + th2B + th3B);
                                                                            cmx];

end
